simulink model "time_frequency_domain"  (R2021a)
settings: Solver=VariableStepAuto  StartTime=0.0  StopTime=5  RelTol=1e-3
libraries: commanapbnd3 x2, dspsrcs4 x2, dspxfrm3 x1
settings Model: Creator=Acer  LastModifiedBy=Acer

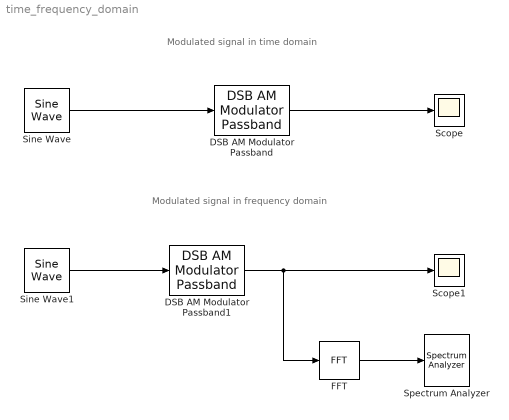
== system time_frequency_domain ==
  note: Modulated signal in time domain
  note: Modulated signal in frequency domain
  DSB AM Modulator Passband : commanapbnd3/DSB AM Modulator Passband  Fc=200  Ph=0  Offset=1
      settings: SourceProductBaseCode=CM
  DSB AM Modulator Passband1 : commanapbnd3/DSB AM Modulator Passband  Fc=200  Ph=0  Offset=1
      settings: SourceProductBaseCode=CM
  FFT : dspxfrm3/FFT  FFTImplementation=Auto  CompMethod=Table lookup  TableOpt=NEW  TableOptActive=Speed  BitRevOrder=off  Normalize=off  InheritFFTLength=on  FFTLength=64  WrapInput=on  roundingMode=Floor  overflowMode=off  firstCoeffDataTypeStr=Inherit: Same word length as input  firstCoeffLastDataTypeStr=Inherit: Same word length as input  outputMin=[]  outputMax=[]
  Scope : Scope
  Scope1 : Scope
  Sine Wave : dspsrcs4/Sine Wave  Amplitude=1  Frequency=10  Phase=0  SampleMode=Discrete  OutComplex=Real  CompMethod=Trigonometric fcn  TableSize=Speed  SampleTime=1/1000  SamplesPerFrame=1  ResetState=Restart at time zero  OutputFrames=off  dataType=double  wordLen=16  udDataType=sfix(16)  fracBitsMode=Best precision  numFracBits=15  OutDataTypeStr=double  LastOutDataTypeStr=double
  Sine Wave1 : dspsrcs4/Sine Wave  Amplitude=1  Frequency=10  Phase=0  SampleMode=Discrete  OutComplex=Real  CompMethod=Trigonometric fcn  TableSize=Speed  SampleTime=1/1000  SamplesPerFrame=1  ResetState=Restart at time zero  OutputFrames=off  dataType=double  wordLen=16  udDataType=sfix(16)  fracBitsMode=Best precision  numFracBits=15  OutDataTypeStr=double  LastOutDataTypeStr=double
  Spectrum Analyzer : SpectrumAnalyzer
  wires:
  Sine Wave/1 -> DSB AM Modulator Passband/1
  DSB AM Modulator Passband/1 -> Scope/1
  Sine Wave1/1 -> DSB AM Modulator Passband1/1
  DSB AM Modulator Passband1/1 -> FFT/1, Scope1/1
  FFT/1 -> Spectrum Analyzer/1
